simulink model "punto_8_3"  (R2023b)
settings: Solver=VariableStepAuto  StartTime=0.0  StopTime=1  RelTol=1e-3
undefined symbols (not defined in the file): C, u_e, x_e
libraries: cstblocks x6
settings Model: Creator=guidocarnevale  LastModifiedBy=lverc

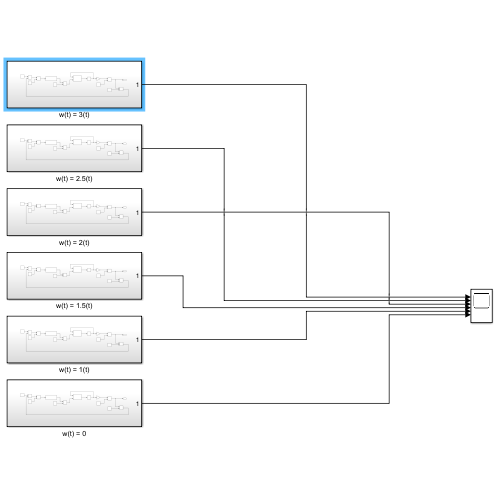
[thumbnail: Simulink's stored preview of the top-level diagram]
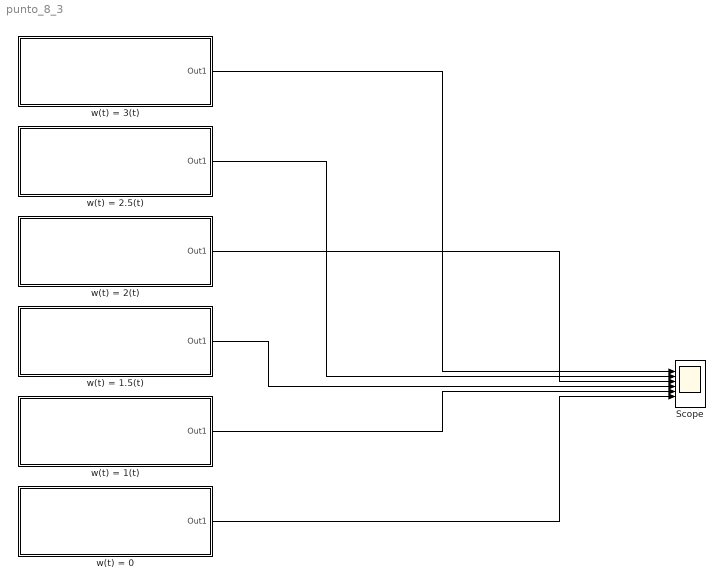
== system punto_8_3 ==
  Scope : Scope  NumInputPorts=6
  w(t) = 0 : Subsystem
  w(t) = 1(t) : Subsystem
  w(t) = 1.5(t) : Subsystem
  w(t) = 2(t) : Subsystem
  w(t) = 2.5(t) : Subsystem
  w(t) = 3(t) : Subsystem
  wires:
  w(t) = 3(t)/1(Out1) -> Scope/1
  w(t) = 2.5(t)/1(Out1) -> Scope/2
  w(t) = 2(t)/1(Out1) -> Scope/3
  w(t) = 1.5(t)/1(Out1) -> Scope/4
  w(t) = 1(t)/1(Out1) -> Scope/5
  w(t) = 0/1(Out1) -> Scope/6

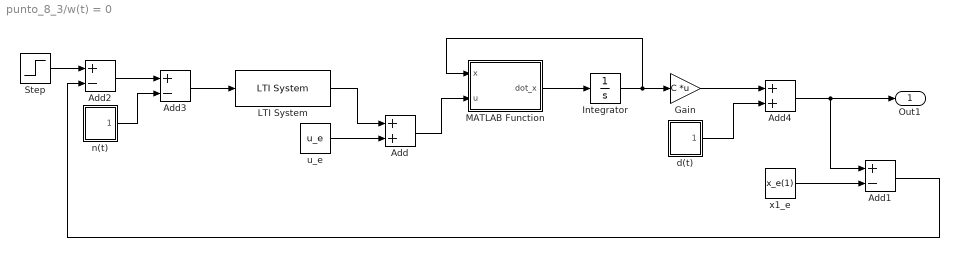
== system punto_8_3/w(t) = 0 ==
  Add : Sum
  Add1 : Sum  Inputs=+-
  Add2 : Sum  Inputs=+-
  Add3 : Sum  Inputs=+-
  Add4 : Sum
  Gain : Gain  Gain=C  Multiplication=Matrix(K*u)
  Integrator : Integrator  InitialCondition=x_e
  LTI System : cstblocks/LTI System  sys=RR  IC=[]  PadeOrder=0
  MATLAB Function : MATLAB Function  TreatAsAtomicUnit=on
  Step : Step  Time=0  After=0  SampleTime=0
  d(t) : Subsystem
  n(t) : Subsystem
  u_e : Constant  Value=u_e
  x1_e : Constant  Value=x_e(1)
  Out1 : Outport
  wires:
  Add3/1 -> LTI System/1
  Gain/1 -> Add4/1
  Add1/1 -> Add2/2
  Add/1 -> MATLAB Function/2(u)
  MATLAB Function/1(dot_x) -> Integrator/1
  Step/1 -> Add2/1
  n(t)/1(" ") -> Add3/2
  Add2/1 -> Add3/1
  x1_e/1 -> Add1/2
  LTI System/1 -> Add/1
  Integrator/1 -> MATLAB Function/1(x), Gain/1
  u_e/1 -> Add/2
  d(t)/1(" ") -> Add4/2
  Add4/1 -> Out1/1, Add1/1

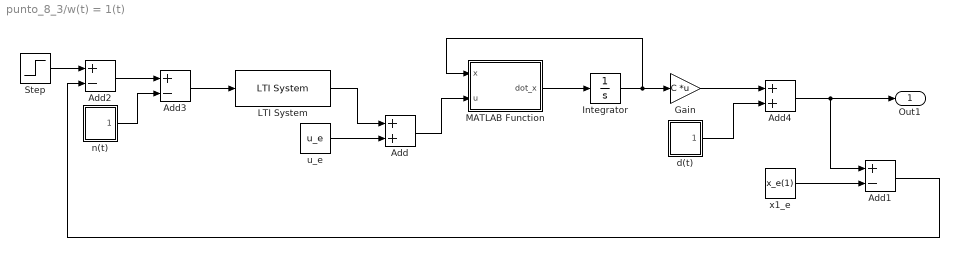
== system punto_8_3/w(t) = 1(t) ==
  Add : Sum
  Add1 : Sum  Inputs=+-
  Add2 : Sum  Inputs=+-
  Add3 : Sum  Inputs=+-
  Add4 : Sum
  Gain : Gain  Gain=C  Multiplication=Matrix(K*u)
  Integrator : Integrator  InitialCondition=x_e
  LTI System : cstblocks/LTI System  sys=RR  IC=[]  PadeOrder=0
  MATLAB Function : MATLAB Function  TreatAsAtomicUnit=on
  Step : Step  Time=0  SampleTime=0
  d(t) : Subsystem
  n(t) : Subsystem
  u_e : Constant  Value=u_e
  x1_e : Constant  Value=x_e(1)
  Out1 : Outport
  wires:
  Add3/1 -> LTI System/1
  Gain/1 -> Add4/1
  Add1/1 -> Add2/2
  Add/1 -> MATLAB Function/2(u)
  MATLAB Function/1(dot_x) -> Integrator/1
  Step/1 -> Add2/1
  n(t)/1(" ") -> Add3/2
  Add2/1 -> Add3/1
  x1_e/1 -> Add1/2
  LTI System/1 -> Add/1
  Integrator/1 -> MATLAB Function/1(x), Gain/1
  u_e/1 -> Add/2
  d(t)/1(" ") -> Add4/2
  Add4/1 -> Out1/1, Add1/1

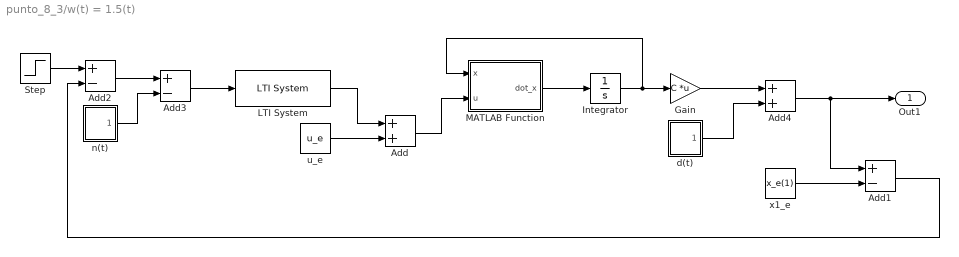
== system punto_8_3/w(t) = 1.5(t) ==
  Add : Sum
  Add1 : Sum  Inputs=+-
  Add2 : Sum  Inputs=+-
  Add3 : Sum  Inputs=+-
  Add4 : Sum
  Gain : Gain  Gain=C  Multiplication=Matrix(K*u)
  Integrator : Integrator  InitialCondition=x_e
  LTI System : cstblocks/LTI System  sys=RR  IC=[]  PadeOrder=0
  MATLAB Function : MATLAB Function  TreatAsAtomicUnit=on
  Step : Step  Time=0  After=1.5  SampleTime=0
  d(t) : Subsystem
  n(t) : Subsystem
  u_e : Constant  Value=u_e
  x1_e : Constant  Value=x_e(1)
  Out1 : Outport
  wires:
  Add3/1 -> LTI System/1
  Gain/1 -> Add4/1
  Add1/1 -> Add2/2
  Add/1 -> MATLAB Function/2(u)
  MATLAB Function/1(dot_x) -> Integrator/1
  Step/1 -> Add2/1
  n(t)/1(" ") -> Add3/2
  Add2/1 -> Add3/1
  x1_e/1 -> Add1/2
  LTI System/1 -> Add/1
  Integrator/1 -> MATLAB Function/1(x), Gain/1
  u_e/1 -> Add/2
  d(t)/1(" ") -> Add4/2
  Add4/1 -> Out1/1, Add1/1

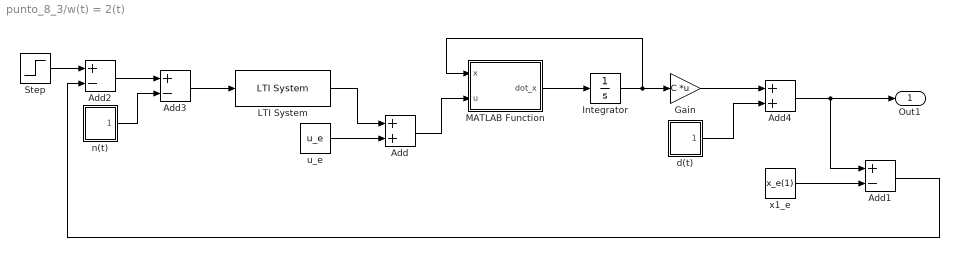
== system punto_8_3/w(t) = 2(t) ==
  Add : Sum
  Add1 : Sum  Inputs=+-
  Add2 : Sum  Inputs=+-
  Add3 : Sum  Inputs=+-
  Add4 : Sum
  Gain : Gain  Gain=C  Multiplication=Matrix(K*u)
  Integrator : Integrator  InitialCondition=x_e
  LTI System : cstblocks/LTI System  sys=RR  IC=[]  PadeOrder=0
  MATLAB Function : MATLAB Function  TreatAsAtomicUnit=on
  Step : Step  Time=0  After=2  SampleTime=0
  d(t) : Subsystem
  n(t) : Subsystem
  u_e : Constant  Value=u_e
  x1_e : Constant  Value=x_e(1)
  Out1 : Outport
  wires:
  Add3/1 -> LTI System/1
  Gain/1 -> Add4/1
  Add1/1 -> Add2/2
  Add/1 -> MATLAB Function/2(u)
  MATLAB Function/1(dot_x) -> Integrator/1
  Step/1 -> Add2/1
  n(t)/1(" ") -> Add3/2
  Add2/1 -> Add3/1
  x1_e/1 -> Add1/2
  LTI System/1 -> Add/1
  Integrator/1 -> MATLAB Function/1(x), Gain/1
  u_e/1 -> Add/2
  d(t)/1(" ") -> Add4/2
  Add4/1 -> Out1/1, Add1/1

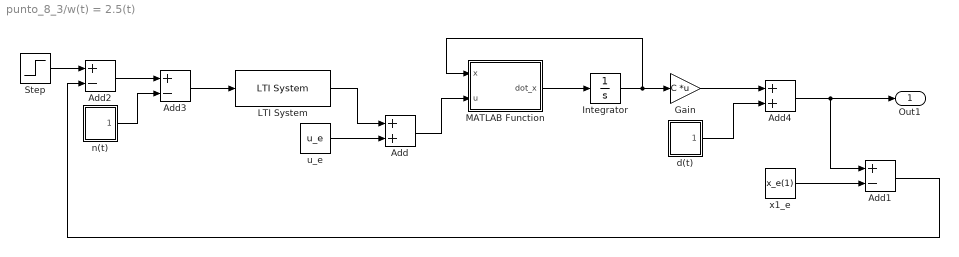
== system punto_8_3/w(t) = 2.5(t) ==
  Add : Sum
  Add1 : Sum  Inputs=+-
  Add2 : Sum  Inputs=+-
  Add3 : Sum  Inputs=+-
  Add4 : Sum
  Gain : Gain  Gain=C  Multiplication=Matrix(K*u)
  Integrator : Integrator  InitialCondition=x_e
  LTI System : cstblocks/LTI System  sys=RR  IC=[]  PadeOrder=0
  MATLAB Function : MATLAB Function  TreatAsAtomicUnit=on
  Step : Step  Time=0  After=2.5  SampleTime=0
  d(t) : Subsystem
  n(t) : Subsystem
  u_e : Constant  Value=u_e
  x1_e : Constant  Value=x_e(1)
  Out1 : Outport
  wires:
  Add3/1 -> LTI System/1
  Gain/1 -> Add4/1
  Add1/1 -> Add2/2
  Add/1 -> MATLAB Function/2(u)
  MATLAB Function/1(dot_x) -> Integrator/1
  Step/1 -> Add2/1
  n(t)/1(" ") -> Add3/2
  Add2/1 -> Add3/1
  x1_e/1 -> Add1/2
  LTI System/1 -> Add/1
  Integrator/1 -> MATLAB Function/1(x), Gain/1
  u_e/1 -> Add/2
  d(t)/1(" ") -> Add4/2
  Add4/1 -> Out1/1, Add1/1

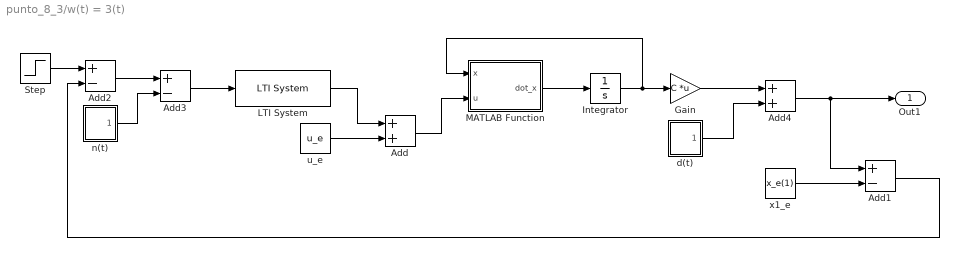
== system punto_8_3/w(t) = 3(t) ==
  Add : Sum
  Add1 : Sum  Inputs=+-
  Add2 : Sum  Inputs=+-
  Add3 : Sum  Inputs=+-
  Add4 : Sum
  Gain : Gain  Gain=C  Multiplication=Matrix(K*u)
  Integrator : Integrator  InitialCondition=x_e
  LTI System : cstblocks/LTI System  sys=RR  IC=[]  PadeOrder=0
  MATLAB Function : MATLAB Function  TreatAsAtomicUnit=on
  Step : Step  Time=0  After=3  SampleTime=0
  d(t) : Subsystem
  n(t) : Subsystem
  u_e : Constant  Value=u_e
  x1_e : Constant  Value=x_e(1)
  Out1 : Outport
  wires:
  Add3/1 -> LTI System/1
  Gain/1 -> Add4/1
  Add1/1 -> Add2/2
  Add/1 -> MATLAB Function/2(u)
  MATLAB Function/1(dot_x) -> Integrator/1
  Step/1 -> Add2/1
  n(t)/1(" ") -> Add3/2
  Add2/1 -> Add3/1
  x1_e/1 -> Add1/2
  LTI System/1 -> Add/1
  Integrator/1 -> MATLAB Function/1(x), Gain/1
  u_e/1 -> Add/2
  d(t)/1(" ") -> Add4/2
  Add4/1 -> Out1/1, Add1/1

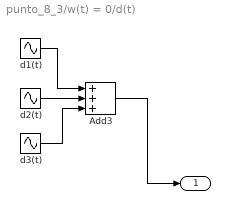
== system punto_8_3/w(t) = 0/d(t) ==
  Add3 : Sum  Inputs=+++
  d1(t) : Sin  Amplitude=3  Frequency=0.01  SampleTime=0
  d2(t) : Sin  Amplitude=3  Frequency=0.01*2  SampleTime=0
  d3(t) : Sin  Amplitude=3  Frequency=0.01*3  SampleTime=0
  " " : Outport
  wires:
  Add3/1 -> " "/1
  d3(t)/1 -> Add3/3
  d1(t)/1 -> Add3/1
  d2(t)/1 -> Add3/2

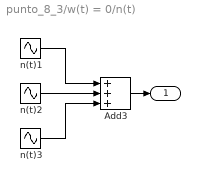
== system punto_8_3/w(t) = 0/n(t) ==
  Add3 : Sum  Inputs=+++
  n(t)1 : Sin  Amplitude=3  Frequency=(10^5)  SampleTime=0
  n(t)2 : Sin  Amplitude=3  Frequency=(10^5)*2  SampleTime=0
  n(t)3 : Sin  Amplitude=3  Frequency=(10^5)*3  SampleTime=0
  " " : Outport
  wires:
  n(t)1/1 -> Add3/1
  n(t)3/1 -> Add3/3
  n(t)2/1 -> Add3/2
  Add3/1 -> " "/1

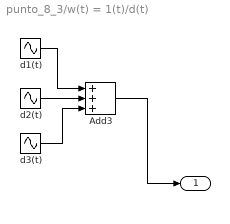
== system punto_8_3/w(t) = 1(t)/d(t) ==
  Add3 : Sum  Inputs=+++
  d1(t) : Sin  Amplitude=3  Frequency=0.01  SampleTime=0
  d2(t) : Sin  Amplitude=3  Frequency=0.01*2  SampleTime=0
  d3(t) : Sin  Amplitude=3  Frequency=0.01*3  SampleTime=0
  " " : Outport
  wires:
  Add3/1 -> " "/1
  d3(t)/1 -> Add3/3
  d1(t)/1 -> Add3/1
  d2(t)/1 -> Add3/2

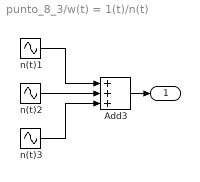
== system punto_8_3/w(t) = 1(t)/n(t) ==
  Add3 : Sum  Inputs=+++
  n(t)1 : Sin  Amplitude=3  Frequency=(10^5)  SampleTime=0
  n(t)2 : Sin  Amplitude=3  Frequency=(10^5)*2  SampleTime=0
  n(t)3 : Sin  Amplitude=3  Frequency=(10^5)*3  SampleTime=0
  " " : Outport
  wires:
  n(t)1/1 -> Add3/1
  n(t)3/1 -> Add3/3
  n(t)2/1 -> Add3/2
  Add3/1 -> " "/1

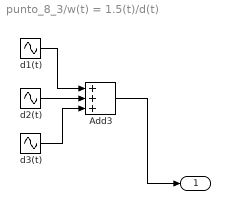
== system punto_8_3/w(t) = 1.5(t)/d(t) ==
  Add3 : Sum  Inputs=+++
  d1(t) : Sin  Amplitude=3  Frequency=0.01  SampleTime=0
  d2(t) : Sin  Amplitude=3  Frequency=0.01*2  SampleTime=0
  d3(t) : Sin  Amplitude=3  Frequency=0.01*3  SampleTime=0
  " " : Outport
  wires:
  Add3/1 -> " "/1
  d3(t)/1 -> Add3/3
  d1(t)/1 -> Add3/1
  d2(t)/1 -> Add3/2

== system punto_8_3/w(t) = 1.5(t)/n(t) ==
  Add3 : Sum  Inputs=+++
  n(t)1 : Sin  Amplitude=3  Frequency=(10^5)  SampleTime=0
  n(t)2 : Sin  Amplitude=3  Frequency=(10^5)*2  SampleTime=0
  n(t)3 : Sin  Amplitude=3  Frequency=(10^5)*3  SampleTime=0
  " " : Outport
  wires:
  n(t)1/1 -> Add3/1
  n(t)3/1 -> Add3/3
  n(t)2/1 -> Add3/2
  Add3/1 -> " "/1

== system punto_8_3/w(t) = 2(t)/d(t) ==
  Add3 : Sum  Inputs=+++
  d1(t) : Sin  Amplitude=3  Frequency=0.01  SampleTime=0
  d2(t) : Sin  Amplitude=3  Frequency=0.01*2  SampleTime=0
  d3(t) : Sin  Amplitude=3  Frequency=0.01*3  SampleTime=0
  " " : Outport
  wires:
  Add3/1 -> " "/1
  d3(t)/1 -> Add3/3
  d1(t)/1 -> Add3/1
  d2(t)/1 -> Add3/2

== system punto_8_3/w(t) = 2(t)/n(t) ==
  Add3 : Sum  Inputs=+++
  n(t)1 : Sin  Amplitude=3  Frequency=(10^5)  SampleTime=0
  n(t)2 : Sin  Amplitude=3  Frequency=(10^5)*2  SampleTime=0
  n(t)3 : Sin  Amplitude=3  Frequency=(10^5)*3  SampleTime=0
  " " : Outport
  wires:
  n(t)1/1 -> Add3/1
  n(t)3/1 -> Add3/3
  n(t)2/1 -> Add3/2
  Add3/1 -> " "/1

== system punto_8_3/w(t) = 2.5(t)/d(t) ==
  Add3 : Sum  Inputs=+++
  d1(t) : Sin  Amplitude=3  Frequency=0.01  SampleTime=0
  d2(t) : Sin  Amplitude=3  Frequency=0.01*2  SampleTime=0
  d3(t) : Sin  Amplitude=3  Frequency=0.01*3  SampleTime=0
  " " : Outport
  wires:
  Add3/1 -> " "/1
  d3(t)/1 -> Add3/3
  d1(t)/1 -> Add3/1
  d2(t)/1 -> Add3/2

== system punto_8_3/w(t) = 2.5(t)/n(t) ==
  Add3 : Sum  Inputs=+++
  n(t)1 : Sin  Amplitude=3  Frequency=(10^5)  SampleTime=0
  n(t)2 : Sin  Amplitude=3  Frequency=(10^5)*2  SampleTime=0
  n(t)3 : Sin  Amplitude=3  Frequency=(10^5)*3  SampleTime=0
  " " : Outport
  wires:
  n(t)1/1 -> Add3/1
  n(t)3/1 -> Add3/3
  n(t)2/1 -> Add3/2
  Add3/1 -> " "/1

== system punto_8_3/w(t) = 3(t)/d(t) ==
  Add3 : Sum  Inputs=+++
  d1(t) : Sin  Amplitude=3  Frequency=0.01  SampleTime=0
  d2(t) : Sin  Amplitude=3  Frequency=0.01*2  SampleTime=0
  d3(t) : Sin  Amplitude=3  Frequency=0.01*3  SampleTime=0
  " " : Outport
  wires:
  Add3/1 -> " "/1
  d3(t)/1 -> Add3/3
  d1(t)/1 -> Add3/1
  d2(t)/1 -> Add3/2

== system punto_8_3/w(t) = 3(t)/n(t) ==
  Add3 : Sum  Inputs=+++
  n(t)1 : Sin  Amplitude=3  Frequency=(10^5)  SampleTime=0
  n(t)2 : Sin  Amplitude=3  Frequency=(10^5)*2  SampleTime=0
  n(t)3 : Sin  Amplitude=3  Frequency=(10^5)*3  SampleTime=0
  " " : Outport
  wires:
  n(t)1/1 -> Add3/1
  n(t)3/1 -> Add3/3
  n(t)2/1 -> Add3/2
  Add3/1 -> " "/1

== matlab function punto_8_3/w(t) = 0/MATLAB Function ==
  data: x input; u input; dot_x output
function dot_x = f(x,u)

%Valori forniti da specifica
beta = 0.2;
k = 20;

J = @(theta) 2+0.5*cos(theta - 1) + 0.5*cos(2*theta +2) + 0.01*cos(3*theta + 1.5) + 0.01*cos(4*theta -2);

dot_x = zeros(2,1);

dot_x(1) = x(2);
dot_x(2) = -beta*x(2)/J(x(1)) + u/J(x(1)) - k*x(1)/J(x(1));

== matlab function punto_8_3/w(t) = 1.5(t)/MATLAB Function ==
  data: x input; u input; dot_x output
function dot_x = f(x,u)

%Valori forniti da specifica
beta = 0.2;
k = 20;

J = @(theta) 2+0.5*cos(theta - 1) + 0.5*cos(2*theta +2) + 0.01*cos(3*theta + 1.5) + 0.01*cos(4*theta -2);

dot_x = zeros(2,1);

dot_x(1) = x(2);
dot_x(2) = -beta*x(2)/J(x(1)) + u/J(x(1)) - k*x(1)/J(x(1));

== matlab function punto_8_3/w(t) = 2(t)/MATLAB Function ==
  data: x input; u input; dot_x output
function dot_x = f(x,u)

%Valori forniti da specifica
beta = 0.2;
k = 20;

J = @(theta) 2+0.5*cos(theta - 1) + 0.5*cos(2*theta +2) + 0.01*cos(3*theta + 1.5) + 0.01*cos(4*theta -2);

dot_x = zeros(2,1);

dot_x(1) = x(2);
dot_x(2) = -beta*x(2)/J(x(1)) + u/J(x(1)) - k*x(1)/J(x(1));

== matlab function punto_8_3/w(t) = 2.5(t)/MATLAB Function ==
  data: x input; u input; dot_x output
function dot_x = f(x,u)

%Valori forniti da specifica
beta = 0.2;
k = 20;

J = @(theta) 2+0.5*cos(theta - 1) + 0.5*cos(2*theta +2) + 0.01*cos(3*theta + 1.5) + 0.01*cos(4*theta -2);

dot_x = zeros(2,1);

dot_x(1) = x(2);
dot_x(2) = -beta*x(2)/J(x(1)) + u/J(x(1)) - k*x(1)/J(x(1));

== matlab function punto_8_3/w(t) = 3(t)/MATLAB Function ==
  data: x input; u input; dot_x output
function dot_x = f(x,u)

%Valori forniti da specifica
beta = 0.2;
k = 20;

J = @(theta) 2+0.5*cos(theta - 1) + 0.5*cos(2*theta +2) + 0.01*cos(3*theta + 1.5) + 0.01*cos(4*theta -2);

dot_x = zeros(2,1);

dot_x(1) = x(2);
dot_x(2) = -beta*x(2)/J(x(1)) + u/J(x(1)) - k*x(1)/J(x(1));

== matlab function punto_8_3/w(t) = 1(t)/MATLAB Function ==
  data: x input; u input; dot_x output
function dot_x = f(x,u)

%Valori forniti da specifica
beta = 0.2;
k = 20;

J = @(theta) 2+0.5*cos(theta - 1) + 0.5*cos(2*theta +2) + 0.01*cos(3*theta + 1.5) + 0.01*cos(4*theta -2);

dot_x = zeros(2,1);

dot_x(1) = x(2);
dot_x(2) = -beta*x(2)/J(x(1)) + u/J(x(1)) - k*x(1)/J(x(1));
